simulink model "newton_raphson"  (R2021a)
settings: Solver=FixedStepDiscrete  StartTime=0.0  StopTime=inf  FixedStep=1  RelTol=1e-3
libraries: simulink x1
settings Model: Creator=manur  LastModifiedBy=manur

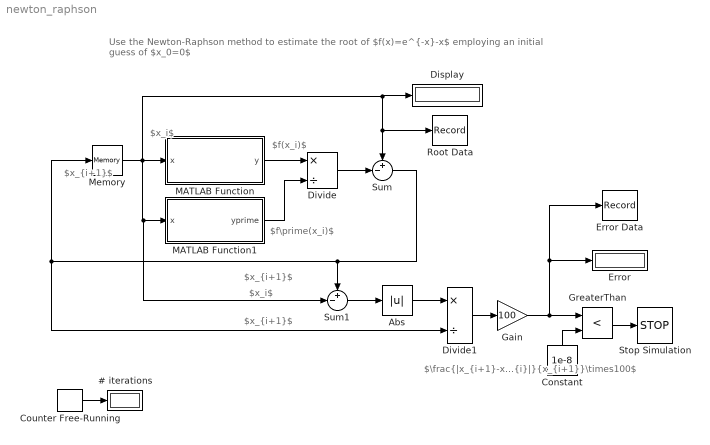
== system newton_raphson ==
  note: $x_i$
  note: $f(x_i)$
  note: Use the Newton-Raphson method to estimate the root of $f(x)=e^{-x}-x$ employing an initial guess of $x_0=0$
  note: $f\prime(x_i)$
  note: $x_{i+1}$
  note: $\frac{|x_{i+1}-x_{i}|}{x_{i+1}}\times100$
  note: $x_{i+1}$
  note: $x_i$
  note: $x_{i+1}$
  # iterations : Display
  Abs : Abs
  Constant : Constant  Value=1e-8
  Counter Free-Running : simulink/Sources/Counter Free-Running  NumBits=16  tsamp=-1
  Display : Display
  Divide : Product  Inputs=*/
  Divide1 : Product  Inputs=*/
  Error : Display
  Error Data : Record  FileSettingsInternal="{\"entries\":[{\"content\":{\"excelSettings\":{\"content\":{},\"type\":\"Streamout.ExcelSettings\"}},\"type\":\"Streamout.FileSettingStorage\",\"uuid\":\"d0b3212f-3a47-45c4-98f1-de8677493811\"}],\"packageUris\":[\"http://schema.mathworks.com/mf0/streamout_blocks/R2020a\"],\"version\":\"1.0\"}"  SignalsInternal="{\"entries\":[{\"content\":{\"signals\":[{\"content\":{\"blockPath\":[\"newton_raphson/Record1\"],\"channel\":[],\"dimensions\":[1],\"domain\":\"newton_raphson/record1\",\"lineColor\":\"#fe330a\",\"plots\":[1],\"port\":1,\"sid\":[\"\"],\"signalID\":265,\"signalName\":\"Gain\"},\"type\":\"RecordBlkView.Signal\",\"uuid\":\"b320e905-fb17-401b-8dcd-666d29ec7e04\"}]},\"type\":\"RecordBlkView.InputSignals\",\"uuid\":\"6273a4fa-21d6-41ce-9b63-6e90cff081b8\"}],\"packageUris\":[\"http://schema.mathworks.com/mf0/streamout_blocks/R2020a\"],\"version\":\"1.0\"}"  VisualizationBindings="{\"sparklinesplugin\":{\"info\":[{\"bindingParametersList\":[],\"subplotID\":1}]}}"
  Gain : Gain  Gain=100
  GreaterThan : RelationalOperator  Operator=<  OutDataTypeStr=boolean  RndMeth=Simplest
  MATLAB Function : MATLAB Function  TreatAsAtomicUnit=on
  MATLAB Function1 : MATLAB Function  TreatAsAtomicUnit=on
  Memory : Memory
  Root Data : Record  FileSettingsInternal="{\"entries\":[{\"content\":{\"excelSettings\":{\"content\":{},\"type\":\"Streamout.ExcelSettings\"}},\"type\":\"Streamout.FileSettingStorage\",\"uuid\":\"51d8a065-b33e-4dc7-a8b0-b2f22ffb6cb9\"}],\"packageUris\":[\"http://schema.mathworks.com/mf0/streamout_blocks/R2020a\"],\"version\":\"1.0\"}"  SignalsInternal="{\"entries\":[{\"content\":{\"signals\":[{\"content\":{\"blockPath\":[\"newton_raphson/Record\"],\"channel\":[],\"dimensions\":[1],\"domain\":\"newton_raphson/record\",\"lineColor\":\"#b746ff\",\"plots\":[1],\"port\":1,\"sid\":[\"\"],\"signalID\":261,\"signalName\":\"Memory\"},\"type\":\"RecordBlkView.Signal\",\"uuid\":\"4fca3a61-f9fb-45bf-8e35-35e257ddf67f\"}]},\"type\":\"RecordBlkView.InputSignals\",\"uuid\":\"db3476f3-ca96-41ec-8447-a9166ac80719\"}],\"packageUris\":[\"http://schema.mathworks.com/mf0/streamout_blocks/R2020a\"],\"version\":\"1.0\"}"  VisualizationBindings="{\"sparklinesplugin\":{\"info\":[{\"bindingParametersList\":[],\"subplotID\":1}]}}"
  Stop Simulation : Stop
  Sum : Sum  Inputs=+-|
  Sum1 : Sum  Inputs=+-|
  wires:
  MATLAB Function/1(y) -> Divide/1
  MATLAB Function1/1(yprime) -> Divide/2
  Divide/1 -> Sum/2
  Memory/1 -> MATLAB Function/1(x), Sum/1, Root Data/1, Display/1, Sum1/2, MATLAB Function1/1(x)
  Sum/1 -> Sum1/1, Divide1/2, Memory/1
  Sum1/1 -> Abs/1
  Divide1/1 -> Gain/1
  Abs/1 -> Divide1/1
  Constant/1 -> GreaterThan/2
  GreaterThan/1 -> Stop Simulation/1
  Gain/1 -> GreaterThan/1, Error/1, Error Data/1
  Counter Free-Running/1 -> # iterations/1

== matlab function newton_raphson/MATLAB Function ==
  data: x input; y output
function y = f(x)

y = exp(-x)-x;

== matlab function newton_raphson/MATLAB Function1 ==
  data: x input; yprime output
function yprime = fprime(x)

yprime = -exp(-x)-1;
